simulink model "controller_v12"  (R2022a)
settings: Solver=FixedStepDiscrete  StartTime=0.0  StopTime=inf  RelTol=1e-3
undefined symbols (not defined in the file): ctr, DiscIntNeverNeededParam, flt, IO397, mdl, rbt, rsim, som, ukf_P0_flat, ukf_prediction_time, ukf_s0, ukf_sys, ukf_use_prediction
libraries: simulink x31, slrealtimeloglib x14, slrealtimetgmanagement x5, slrealtimeseriallib x5, speedgoatlib_fpga_analog_io x4, speedgoatlib_fpga x2, speedgoatlib_fpga_dio x1, slrealtimeutilitieslib x1
(part 4 of 4)

== matlab function controller_v12/Adaptive Controller/attitude and thrust MPC controller/MATLAB Function ==
  data: Tx input; Tx_out output; Ty input; time input; Ty_out output; mdl parameter; ctr parameter
function [Tx_out, Ty_out] = fcn(Tx, Ty, time, mdl, ctr)

if time > mdl.i_delay && ctr.en
    Tx_out = Tx;
    Ty_out = Ty;
else
    Tx_out = 0;
    Ty_out = 0;
end

end

== matlab function controller_v12/Adaptive Controller/observer/ICRA'23/lateral KF observer/Translational Dynamics & Kinamatics Lin Obs ==
  data: R input; pos_hat output; f_cmd input; meas_pos input; pos_hat input; vel_hat input; vel_hat output; ctr parameter; rbt parameter; acc_hat output; mdl parameter; id_in input; id_out output
function [pos_hat, vel_hat, acc_hat, id_out] = fcn(R, f_cmd, meas_pos, pos_hat, vel_hat, ctr, rbt, mdl, id_in)


pos_hat = pos_hat(:);
vel_hat = vel_hat(:);
meas_pos = meas_pos(:);
R11 = R(1);
R12 = R(2);
R13 = R(3);
R21 = R(4);
R22 = R(5);
R23 = R(6);
R31 = R(7);
R32 = R(8);
R33 = R(9);
R1 = [R11; R21; R31];     % unit (column) vector
R2 = [R12; R22; R32];
R3 = [R13; R23; R33];
R = [R1, R2, R3];



if ctr.en
    u = (R*[0; 0; f_cmd] - [0; 0; rbt.m*mdl.g])/rbt.m;
else
    u = [0; 0; 0]; 
end

u = (R*[0; 0; f_cmd] - [0; 0; rbt.m*mdl.g])/rbt.m;
x_hat_curr = [pos_hat(:); vel_hat(:)];
y = meas_pos; 
x_hat_pred = ctr.pos_vel_est.A*x_hat_curr + ctr.pos_vel_est.B(:, 1:3)*u; 
x_hat_next = (x_hat_pred + ctr.pos_vel_est.L*(y - ctr.pos_vel_est.C*x_hat_pred));
pos_hat = x_hat_next(1:3);
vel_hat = x_hat_next(4:6);
acc_hat = u;

if id_in < 4
    pos_hat = meas_pos;
end

id_out = id_in + 1;

end

== matlab function controller_v12/Adaptive Controller/observer/observer/UKF1/R_flat to quat ==
  data: R_flat input; q output
function q = fcn(R_flat)
% convertion from rotation matrix to quaternion
q = rotm2quat(UKF.unflatten_matrix(R_flat))';
end

== matlab function controller_v12/Adaptive Controller/observer/observer/UKF1/UKF_inner/UKF update then predict ==
  data: s_out output; z_raw input; z_raw_prev input; f_cmd input; tau_cmd_x input; tau_cmd_y input; s_in input; P_in_flat input; is_init_in input; s_prediction_time input; sys parameter; P_out_flat output; is_init_out output; s_out_pre output; s_prediction_out output
function [s_out, P_out_flat, is_init_out, s_out_pre, s_prediction_out] = fcn(z_raw, z_raw_prev, f_cmd, tau_cmd_x, tau_cmd_y, s_in, P_in_flat, is_init_in, s_prediction_time, sys)
    [s_out, P_out_flat, is_init_out, s_out_pre, s_prediction_out] = UKF.inner_helper(z_raw, z_raw_prev, f_cmd, tau_cmd_x, tau_cmd_y, s_in, P_in_flat, is_init_in, s_prediction_time, sys);
end

== matlab function controller_v12/Adaptive Controller/observer/observer/UKF/UKF_inner/UKF update then predict ==
  data: s_out output; z_raw input; z_raw_prev input; f_cmd input; tau_cmd_x input; tau_cmd_y input; s_in input; P_in_flat input; is_init_in input; sys parameter; P_out_flat output; is_init_out output
function [s_out, P_out_flat, is_init_out] = fcn(z_raw, z_raw_prev, f_cmd, tau_cmd_x, tau_cmd_y, s_in, P_in_flat, is_init_in, sys)
    [s_out, P_out_flat, is_init_out] = UKF.inner_helper(z_raw, z_raw_prev, f_cmd, tau_cmd_x, tau_cmd_y, s_in, P_in_flat, is_init_in, sys);
end

== matlab function controller_v12/Adaptive Controller/attitude and thrust controller1/Attitude Controleller ==
  data: r input; torque_x output size=1; r_dot input; r_dotdot input; R input; Omega input; rd input; rd_d input; rd_dd input; rd_ddd input; rd_dddd input; int_e input; ctr parameter; rbt parameter; torque_y output size=1; torque_z output size=1; att_e output size=3; mdl parameter
 function [torque_x, torque_y, torque_z, att_e] = fcn(r, r_dot, r_dotdot, R, Omega, rd,rd_d,rd_dd,rd_ddd,rd_dddd, int_e, ctr, rbt, mdl)
%#codegen

%% init
R11 = R(1);
R12 = R(2);
R13 = R(3);
R21 = R(4);
R22 = R(5);
R23 = R(6);
R31 = R(7);
R32 = R(8);
R33 = R(9);
R1 = [R11; R21; R31];     % unit (column) vector
R2 = [R12; R22; R32];
R3 = [R13; R23; R33];
wx = Omega(1);
wy = Omega(2);
wz = Omega(3);

Dr = r-rd;
Dr_dot = r_dot-rd_d;

torque_x = -dot(R2,rd_dddd) - ...
    ctr.gain.at3*( mdl.g*wx+dot(R2,rd_ddd) ) - ...
    ctr.gain.at2*( dot(R2,mdl.g*[0;0;1]+rd_dd) ) + ...
    ctr.gain.at1*( dot(R2,Dr_dot) ) + ...
    ctr.gain.at0*( dot(R2,Dr) ) + ...
    ctr.gain.ati*( int_e(1) );
torque_x = torque_x*rbt.ixx/mdl.g;

torque_y = dot(R1,rd_dddd) - ...
    ctr.gain.at3*( mdl.g*wy-dot(R1,rd_ddd) ) - ...
    ctr.gain.at2*( dot(R1,-mdl.g*[0;0;1]-rd_dd) ) - ...
    ctr.gain.at1*( dot(R1,Dr_dot) ) - ...
    ctr.gain.at0*( dot(R1,Dr) ) + ...
    ctr.gain.ati*( int_e(2) );

torque_y = torque_y*rbt.iyy/mdl.g;

torque_z = 0;           % no yaw control

att_e = -[-dot(R2,Dr);dot(R1,Dr);0];

== matlab function controller_v12/Adaptive Controller/observer/observer/UKF/euler to quat ==
  data: euler_angles input; q output
function q = fcn(euler_angles)
% convertion from euler to R block

eu_x = euler_angles(1);
eu_y = euler_angles(2);
eu_z = euler_angles(3);

R = [cos(eu_y)*cos(eu_z); -cos(eu_y)*sin(eu_z); sin(eu_y); ...
    cos(eu_x)*sin(eu_z)+sin(eu_x)*sin(eu_y)*cos(eu_z); cos(eu_x)*cos(eu_z)-sin(eu_x)*sin(eu_y)*sin(eu_z); -sin(eu_x)*cos(eu_y); ...
    sin(eu_x)*sin(eu_z)-cos(eu_x)*sin(eu_y)*cos(eu_z); sin(eu_x)*cos(eu_z)+cos(eu_x)*sin(eu_y)*sin(eu_z); cos(eu_x)*cos(eu_y)];
% R is 1x9

R_unflattened = UKF.unflatten_matrix(R);
q = rotm2quat(R_unflattened)';
      


end

== matlab function controller_v12/Adaptive Controller/observer/observer/UKF/quaternion to rotation matrix ==
  data: q input; R_flat output
function R_flat = fcn(q)
    % Assume q = [q_s; q_x, q_y, q_z];
    R = quat2rotm(q');
    R_flat = UKF.flatten_matrix(R);
end

== matlab function controller_v12/Adaptive Controller/observer/observer/UKF1/pack measurement vector ==
  data: r input; z_raw output; q input
function z_raw = fcn(r, q)
    z_raw = vertcat(r, q, zeros(6,1));
end

== matlab function controller_v12/Adaptive Controller/observer/observer/UKF1/quaternion to rotation matrix ==
  data: q input; R_flat output
function R_flat = fcn(q)
    % Assume q = [q_s; q_x, q_y, q_z];
    R = quat2rotm(q');
    R_flat = UKF.flatten_matrix(R);
end

== matlab function controller_v12/Adaptive Controller/attitude and thrust MPC controller2/MATLAB Function1 ==
  data: u input; y output
function y = fcn(u)

y = u;

== matlab function controller_v12/Adaptive Controller/attitude and thrust MPC controller2/NN RTMPC/MATLAB Function ==
  data: time input; x_in output; r input; r_dot input; r_dotdot input; R input; Omega input; rd input; rd_d input; rd_dd input; rd_ddd input; rd_dddd input; int_e input; mdl parameter; rbt parameter; ctr parameter
function x_in    = fcn(time, r, r_dot, r_dotdot, R, Omega, rd,rd_d,rd_dd,rd_ddd,rd_dddd, int_e, mdl, rbt, ctr)
    %#codegen
    % r: curr pos
    % r_dot: curr vel
    % R: current attitude
    % Omega: current body rates
    % rd : des pos
    % rd_d: des vel
    %% Out: 
    % cmd_B_thrust_z is thrust force on z axis in body (B) frame [N]
    
    % Ensure signals have expected shape
    R11 = R(1);
    R12 = R(2);
    R13 = R(3);
    R21 = R(4);
    R22 = R(5);
    R23 = R(6);
    R31 = R(7);
    R32 = R(8);
    R33 = R(9);
    R1 = [R11; R21; R31];     % unit (column) vector
    R2 = [R12; R22; R32];
    R3 = [R13; R23; R33];
    R = [R1, R2, R3];

    r = r(:);           % position
    r_dot = r_dot(:);   % velocity 

    rd = rd(:);         % desired position
    rd_d = rd_d(:);     % desired velocity
    
    % Compute current attitude as euler angles (:( )
    B_ypr = rotm2eul(R);
    B_est_roll = B_ypr(3);
    B_est_pitch = B_ypr(2);
    B_est_yaw = B_ypr(1);

    % Conver attitude in yaw-invariant frame. 
    B_R_yaw_I = get_B_R_yaw_I(B_est_yaw);
    I_rp = B_R_yaw_I'*[B_est_roll; B_est_pitch];

    % Set reference 
    x_ref_t0 = [rd; rd_d;]; % no attitude feed-forward at the moment. 
    x_ref = repmat(x_ref_t0, 20, 1);
    %mpc.set_reference_trajectory(x_ref);
    
    % Set current state
    x = [r; r_dot; I_rp(1); I_rp(2)];

    x_in = [x; x_ref];
    x_in = x_in(:); % column vector
    
end

function [R] = get_B_R_yaw_I(yaw)
    R = [cos(yaw), sin(yaw); -sin(yaw), cos(yaw)];
end

== matlab function controller_v12/Adaptive Controller/attitude and thrust MPC controller2/NN RTMPC/MATLAB Function1 ==
  data: u_nn input; Rd output; Omegad output; cmd_B_acc_z output; alt_e output; R input; rbt input; mdl input
function [Rd, Omegad, cmd_B_acc_z, alt_e] = fcn(u_nn, R, rbt, mdl)
    %#codegen
    % r: curr pos
    % r_dot: curr vel
    % R: current attitude
    % Omega: current body rates
    % rd : des pos
    % rd_d: des vel
    %% Out: 
    % cmd_B_thrust_z is thrust force on z axis in body (B) frame [N]
    
    % Ensure signals have expected shape
    R11 = R(1);
    R12 = R(2);
    R13 = R(3);
    R21 = R(4);
    R22 = R(5);
    R23 = R(6);
    R31 = R(7);
    R32 = R(8);
    R33 = R(9);
    R1 = [R11; R21; R31];     % unit (column) vector
    R2 = [R12; R22; R32];
    R3 = [R13; R23; R33];
    R = [R1, R2, R3];

    u_nn = u_nn(:);
    
    % Compute current attitude as euler angles (:( )
    B_ypr = rotm2eul(R);
    B_est_roll = B_ypr(3);
    B_est_pitch = B_ypr(2);
    B_est_yaw = B_ypr(1);

    % Conver attitude in yaw-invariant frame. 
    B_R_yaw_I = get_B_R_yaw_I(B_est_yaw);
    I_rp = B_R_yaw_I'*[B_est_roll; B_est_pitch];
    
    delta_cmd_I_roll =  u_nn(1);
    delta_cmd_I_pitch = u_nn(2);
    delta_cmd_I_acc_z = u_nn(3);
    
    % Compensate thrust
    cmd_B_thrust = compensate_thrust(delta_cmd_I_acc_z, B_ypr, rbt.m, mdl.g);
    cmd_B_thrust_z = cmd_B_thrust(3);
    cmd_B_acc_z = cmd_B_thrust_z/rbt.m;
    
    % De-rotate attitude commands in body frame
    cmd_I_rp = [delta_cmd_I_roll; delta_cmd_I_pitch];
    B_R_yaw_I = get_B_R_yaw_I(B_est_yaw);
    cmd_B_rp = B_R_yaw_I*cmd_I_rp;
    
    % Compensate attitude
    [cmd_B_roll, cmd_B_pitch] = compensate_attitude(cmd_B_thrust, cmd_B_rp(1), cmd_B_rp(2), rbt.m, mdl.g);

    % Desired angular velocity
    Omegad = [0.0, 0.0, 0.0]; % TODO

    cmd_B_roll  = cmd_B_rp(1); 
    cmd_B_pitch = cmd_B_rp(2);
    cmd_B_yaw = 0.0*B_est_yaw;

    % Altitude error
    alt_e = r(3) - rd(3); 
    
    % Desired attitude as rotation matrix
    Rd_tmp = eul2rotm([cmd_B_yaw, cmd_B_pitch, cmd_B_roll]);

    
%     %%% TODO: Andrea: remove
%     % Try flip
%     speedf = 5.0;
%     if (time > 1.0) && (time < (1.0 + 1.0/speedf))
%         Rd_tmp = axang2rotm([-1, 0, 0, speedf*2.0*pi*(1.0 - time)]);
%         Omegad = [speedf*2.0*pi, 0.0, 0.0];
%     end
%     %%% 

    % Generate output. 
    Rd_tmp = Rd_tmp'; % this is needed to respect existing convention that rot. matrices are passed
          % around as vectors, created by concatenating the rows of the
          % matrix (and Rd(:) will created a vector by concatentatig the columns of Rd)
    Rd = Rd_tmp(:);
end

function [B_thrust] = compensate_thrust(cmd_B_acc_z, B_ypr, mass, g)
    B_thrust_z = mass * (cmd_B_acc_z+g)/cos(B_ypr(3))/cos(B_ypr(2));
    B_thrust = [0.0; 0.0; B_thrust_z];
end

function [B_roll, B_pitch] = compensate_attitude(B_thrust, lin_B_roll, lin_B_pitch, mass, g)
    B_acc_z = (B_thrust(3))/mass;
    B_roll = lin_B_roll*(g/B_acc_z);
    B_pitch = lin_B_pitch*(g/B_acc_z);
end

function [R] = get_B_R_yaw_I(yaw)
    R = [cos(yaw), sin(yaw); -sin(yaw), cos(yaw)];
end

== matlab function controller_v12/Adaptive Controller/attitude and thrust MPC controller2/NN RTMPC/MATLAB Function2 ==
  data: x input; y output; nnparam parameter
function y = fcn(x, nnparam)
    y = rtmpcnn(x, nnparam)
end

== matlab function controller_v12/Adaptive Controller/attitude and thrust MPC controller2/RTMPC Trajectory Tracking ==
  data: time input; r input; Rd output; r_dot input; r_dotdot input; R input; Omega input; rd input; rd_d input; rd_dd input; rd_ddd input; rd_dddd input; int_e input; ctr parameter; rbt parameter; Omegad output; cmd_B_acc_z output; mdl parameter; alt_e output; rd_rtmpc output
function [Rd, Omegad, cmd_B_acc_z, alt_e, rd_rtmpc]   = fcn(time, r, r_dot, r_dotdot, R, Omega, rd,rd_d,rd_dd,rd_ddd,rd_dddd, int_e, ctr, rbt, mdl)
    %#codegen
    % r: curr pos
    % r_dot: curr vel
    % R: current attitude
    % Omega: current body rates
    % rd : des pos
    % rd_d: des vel
    %% Out: 
    % cmd_B_thrust_z is thrust force on z axis in body (B) frame [N]
    
    % Ensure signals have expected shape
    R11 = R(1);
    R12 = R(2);
    R13 = R(3);
    R21 = R(4);
    R22 = R(5);
    R23 = R(6);
    R31 = R(7);
    R32 = R(8);
    R33 = R(9);
    R1 = [R11; R21; R31];     % unit (column) vector
    R2 = [R12; R22; R32];
    R3 = [R13; R23; R33];
    R = [R1, R2, R3];

    r = r(:);           % position
    r_dot = r_dot(:);   % velocity 

    rd = rd(:);         % desired position
    rd_d = rd_d(:);     % desired velocity
    
    % Compute current attitude as euler angles (:( )
    B_ypr = rotm2eul(R);
    B_est_roll = B_ypr(3);
    B_est_pitch = B_ypr(2);
    B_est_yaw = B_ypr(1);

    % Conver attitude in yaw-invariant frame. 
    B_R_yaw_I = get_B_R_yaw_I(B_est_yaw);
    I_rp = B_R_yaw_I'*[B_est_roll; B_est_pitch];

    % Set reference 
    x_ref = [rd; rd_d; 0.0; 0.0]; % no attitude feed-forward at the moment. 
    %mpc.set_reference_trajectory(x_ref);
    
    % Compute new linearized commands
    x = [r; r_dot; I_rp(1); I_rp(2)];

    % Generate reference % (currently only circle is supported)
    x_ref = traj_planner(time, ctr.rtmpc.ref_len, ctr.rtmpc.traj);

    % Set current state
    x = [r - ctr.rtmpc.r_origin; r_dot; I_rp(1); I_rp(2)];

    if ctr.rtmpc.en
        % Set reference - constant
        % x_ref_t0 = [rd - ctr.rtmpc.r_origin; rd_d;]; % no attitude feed-forward at the moment. 
        % x_ref = repmat(x_ref_t0, 20, 1);

        % Set reference - circle
        % Apply state and reference scaling
        x_scaled = ctr.rtmpc.in_scaling.*x;
        x_ref_scaled = repmat(ctr.rtmpc.in_scaling(1:6), ctr.rtmpc.ref_len, 1).*x_ref;
        
        x_in = [x_scaled; x_ref_scaled];
        x_in = x_in(:); % column vector

        % 10.0 and 12.0 are some scalings applied to the NN to
        % ensure that its input/ouput is in [-1, 1]. 
        % For the rtmpc expert we do not have this care -- but we scale
        % things to ensure that input/outpurs are not too large numbers (e.g., <+-100)
        u_next = 12.0*rtmpcnn(x_in/10.0, ctr.rtmpc.nnparam);

        % Apply rtmpc scaling: 
        u_next = u_next.*ctr.rtmpc.out_scaling;

    else
        x_scaled = x.*ctr.lqr.in_scaling;
        x_ref_scaled = [x_ref(1:6); 0.0; 0.0].*ctr.lqr.in_scaling;
        u_next = -ctr.lqr.K*(x_scaled - x_ref_scaled);
        u_next = u_next.*ctr.lqr.out_scaling;
    end

    rd_rtmpc = x_ref(1:6);
    
    delta_cmd_I_roll =  u_next(1);
    delta_cmd_I_pitch = u_next(2);
    delta_cmd_I_acc_z = u_next(3);
    
    % Compensate thrust
    cmd_B_thrust = compensate_thrust(delta_cmd_I_acc_z, B_ypr, rbt.m, mdl.g);
    cmd_B_thrust_z = cmd_B_thrust(3);
    cmd_B_acc_z = cmd_B_thrust_z/rbt.m;
   
    % apply saturation
    cmd_B_acc_z = max(min(cmd_B_acc_z, mdl.g*1.4), mdl.g*0.7);
    
    % De-rotate attitude commands in body frame
    cmd_I_rp = [delta_cmd_I_roll; delta_cmd_I_pitch];
    B_R_yaw_I = get_B_R_yaw_I(B_est_yaw);
    cmd_B_rp = B_R_yaw_I*cmd_I_rp;
    
    % Compensate attitude
    [cmd_B_roll, cmd_B_pitch] = compensate_attitude(cmd_B_thrust, cmd_B_rp(1), cmd_B_rp(2), rbt.m, mdl.g);
    cmd_B_roll = max(min(cmd_B_roll, ctr.rtmpc.lim.att), -ctr.rtmpc.lim.att);
    cmd_B_pitch = max(min(cmd_B_pitch, ctr.rtmpc.lim.att), -ctr.rtmpc.lim.att);
    cmd_B_yaw = B_est_yaw;

    % Desired angular velocity
    Omegad = [0.0, 0.0, 0.0]; % TODO

    % Altitude error
    alt_e = r(3) - rd(3); 
    
    % Desired attitude as rotation matrix
    Rd_tmp = eul2rotm([cmd_B_yaw, cmd_B_pitch, cmd_B_roll]);

    
%     %%% TODO: Andrea: remove
%     % Try flip
%     speedf = 5.0;
%     if (time > 1.0) && (time < (1.0 + 1.0/speedf))
%         Rd_tmp = axang2rotm([-1, 0, 0, speedf*2.0*pi*(1.0 - time)]);
%         Omegad = [speedf*2.0*pi, 0.0, 0.0];
%     end
%     %%% 

    % Generate output. 
    Rd_tmp = Rd_tmp'; % this is needed to respect existing convention that rot. matrices are passed
          % around as vectors, created by concatenating the rows of the
          % matrix (and Rd(:) will created a vector by concatentatig the columns of Rd)
    Rd = Rd_tmp(:);
end

function [B_thrust] = compensate_thrust(cmd_B_acc_z, B_ypr, mass, g)
    B_thrust_z = mass * (cmd_B_acc_z+g)/cos(B_ypr(3))/cos(B_ypr(2));
    B_thrust = [0.0; 0.0; B_thrust_z];
end

function [B_roll, B_pitch] = compensate_attitude(B_thrust, lin_B_roll, lin_B_pitch, mass, g)
    B_acc_z = (B_thrust(3))/mass;
    B_roll = lin_B_roll*(g/B_acc_z);
    B_pitch = lin_B_pitch*(g/B_acc_z);
end

function [R] = get_B_R_yaw_I(yaw)
    R = [cos(yaw), sin(yaw); -sin(yaw), cos(yaw)];
end

== matlab function controller_v12/Adaptive Controller/attitude and thrust MPC controller2/Rotm2rpy ==
  data: R input; rpy output size=3
function rpy  = fcn(R)
    R = get_rotation_matrix(R);
    ypr = rotm2eul(R); 
    rpy = squeeze([ypr(3); ypr(2); ypr(1)]);

end

function R = get_rotation_matrix(R)
    R11 = R(1);
    R12 = R(2);
    R13 = R(3);
    R21 = R(4);
    R22 = R(5);
    R23 = R(6);
    R31 = R(7);
    R32 = R(8);
    R33 = R(9);
    R1 = [R11; R21; R31];     % unit (column) vector
    R2 = [R12; R22; R32];
    R3 = [R13; R23; R33];
    R = [R1, R2, R3];
end

== matlab function controller_v12/Adaptive Controller/attitude and thrust MPC controller2/Rotm2rpy1 ==
  data: R input; rpy output size=3
function rpy   = fcn(R)
    R = get_rotation_matrix(R);
    ypr = rotm2eul(R); 
    rpy = [ypr(3); ypr(2); ypr(1)];
end

function R = get_rotation_matrix(R)
    R11 = R(1);
    R12 = R(2);
    R13 = R(3);
    R21 = R(4);
    R22 = R(5);
    R23 = R(6);
    R31 = R(7);
    R32 = R(8);
    R33 = R(9);
    R1 = [R11; R21; R31];     % unit (column) vector
    R2 = [R12; R22; R32];
    R3 = [R13; R23; R33];
    R = [R1, R2, R3];
end

== matlab function controller_v12/Adaptive Controller/observer/observer/UKF1/UKF_inner/bee units to SI ==
  data: s_bee input; s_si output
function s_si  = fcn(s_bee)
    s_si = UKF.s_bee_to_s_si(s_bee);
end

== matlab function controller_v12/Adaptive Controller/observer/observer/UKF/pack measurement vector ==
  data: r input; z_raw output; q input; r_dot input; omega input
function z_raw = fcn(r, q, r_dot, omega)
    z_raw = vertcat(r, q, r_dot, omega);
end

== matlab function controller_v12/Adaptive Controller/observer/observer/UKF/unpack state vector ==
  data: s input; r output; q output; r_dot output; omega output
function [r, q, r_dot, omega] = fcn(s)
    [r, q, r_dot, omega] = UKF.partial_unpack_s(s);
end

== matlab function controller_v12/Adaptive Controller/observer/observer/UKF1/UKF_inner/bee cov to SI cov ==
  data: P_flat_bee input; P_flat_si output
function P_flat_si  = fcn(P_flat_bee)
    P_flat_si = UKF.flatten_matrix(diag(UKF.var_bee_to_var_si(diag(UKF.unflatten_matrix(P_flat_bee)))));
end

== matlab function controller_v12/Adaptive Controller/observer/observer/UKF1/UKF_inner/bee units to SI1 ==
  data: s_bee input; s_si output
function s_si  = fcn(s_bee)
    s_si = UKF.s_bee_to_s_si(s_bee);
end

== matlab function controller_v12/Adaptive Controller/observer/observer/UKF1/unpack state ==
  data: s input; r output; q output; r_dot output; omega output
function [r, q, r_dot, omega] = fcn(s)
    [r, q, r_dot, omega, ~, ~] = UKF.unpack_s(s);
end

== matlab function controller_v12/Measurement manager/safety check system/landing condition/landing_cond ==
  data: alt input; en output; time_cond input; ctr parameter
function en = fcn(alt,time_cond,ctr)
%#codegen
if ( (time_cond<0) | (alt>ctr.landing.height) )
    en = 1;
else
    en = 0;
end
en=1;
end
% this lands the robot if the flight time is more than mdl.i_delay+2 and
% the robot is still on the ground.

== matlab function controller_v12/Adaptive Controller/observer/ICRA'23/Rotaion/Rotation Matrix ==
  data: euler_angles input; R output
function R = fcn(euler_angles)
%#codegen

eu_x = euler_angles(1);
eu_y = euler_angles(2);
eu_z = euler_angles(3);

R = [cos(eu_y)*cos(eu_z); -cos(eu_y)*sin(eu_z); sin(eu_y); ...
    cos(eu_x)*sin(eu_z)+sin(eu_x)*sin(eu_y)*cos(eu_z); cos(eu_x)*cos(eu_z)-sin(eu_x)*sin(eu_y)*sin(eu_z); -sin(eu_x)*cos(eu_y); ...
    sin(eu_x)*sin(eu_z)-cos(eu_x)*sin(eu_y)*cos(eu_z); sin(eu_x)*cos(eu_z)+cos(eu_x)*sin(eu_y)*sin(eu_z); cos(eu_x)*cos(eu_y)];
% R is 1x9

== matlab function controller_v12/Adaptive Controller/attitude and thrust controller1/Thrust Controller ==
  data: r input; F output size=1; r_dot input; r_dotdot input; R input; Omega input; rd input; rd_d input; rd_dd input; rd_ddd input; rd_dddd input; int_e input; mdl parameter; alt_e output size=1; ctr parameter
function [F, alt_e] = fcn(r, r_dot, r_dotdot, R, Omega, rd,rd_d,rd_dd,rd_ddd,rd_dddd, int_e, mdl, ctr)
%#codegen

%% init
R11 = R(1);
R12 = R(2);
R13 = R(3);
R21 = R(4);
R22 = R(5);
R23 = R(6);
R31 = R(7);
R32 = R(8);
R33 = R(9);


F = rd_dd(3) - ctr.gain.al1*( r_dot(3)-rd_d(3) ) - ctr.gain.al0*( r(3)-rd(3) );
% F = 0 - ctr.gain.al1*( r_dot(3)) - ctr.gain.al0*( r(3)-ctr.setpoint.z );
F = mdl.g + F + ctr.gain.ali*int_e(4);
F = F/R33;
F = max(min(F, mdl.g+4), mdl.g-3.0); % during hovering.

alt_e = -( r(3)-rd(3) )/R33;
% alt_e = -( r(3)- ctr.setpoint.z )/R33;
end
